simulink model "pv_array"  (R2021a)
settings: Solver=VariableStepAuto  StartTime=0.0  StopTime=10.0  RelTol=1e-3
libraries: spsSeriesRLCBranchLib x2, spsCurrentMeasurementLib x1, spsControlledCurrentSourceLib x1, spsVoltageMeasurementLib x1
settings Model: Creator=Vaneebun  LastModifiedBy=Dell

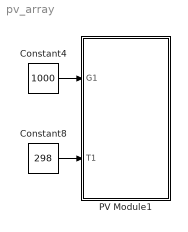
== system pv_array ==
  Constant4 : Constant  Value=1000
  Constant8 : Constant  Value=298
  PV Module1 : Subsystem
  wires:
  Constant8/1 -> PV Module1/2(T1)
  Constant4/1 -> PV Module1/1(G1)

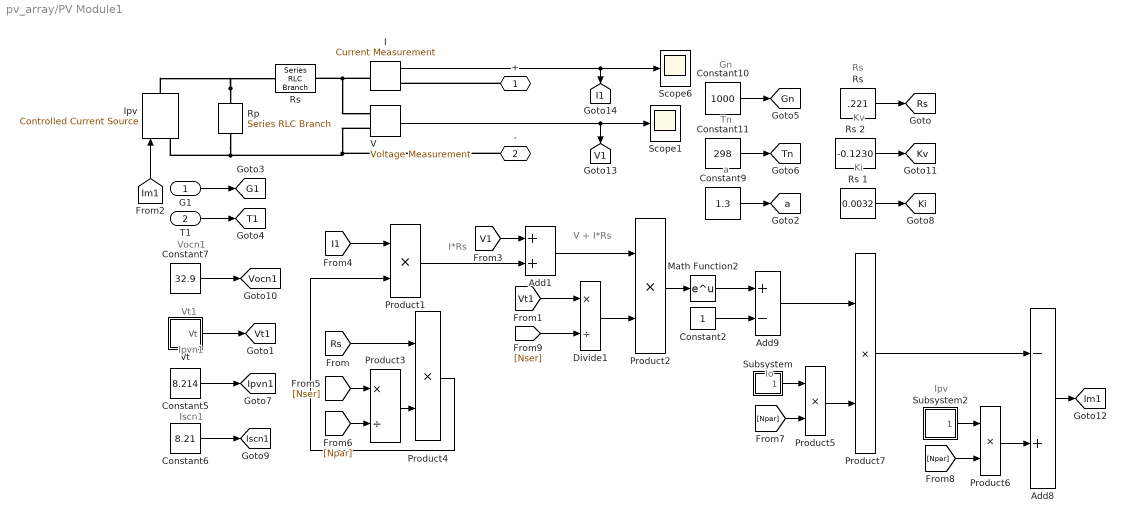
== system pv_array/PV Module1 ==
  note: Vocn1
  note: Iscn1
  note: Ipvn1
  note: I*Rs
  note: Vt1
  note: V + I*Rs
  note: Io
  note: Kv
  note: Ki
  note: Tn
  note: Gn
  note: Rs
  note: a
  note: Ipv
  G1 : Inport
  T1 : Inport  Port=2
  Add1 : Sum
  Add8 : Sum  Inputs=-+
  Add9 : Sum  Inputs=+-
  Constant10 : Constant  Value=1000
  Constant11 : Constant  Value=298
  Constant2 : Constant
  Constant5 : Constant  Value=8.214
  Constant6 : Constant  Value=8.21
  Constant7 : Constant  Value=32.9
  Constant9 : Constant  Value=1.3
  Divide1 : Product  Inputs=*/
  I : spsCurrentMeasurementLib/Current Measurement  PhasorSimulation=off  OutputType=Complex  PSBequivalent=0
  Ipv : spsControlledCurrentSourceLib/Controlled Current Source  Initialize=on  Source_Type=DC  Amplitude=0  Phase=0  Frequency=0  Measurements=None
  Math Function2 : Math  SignedPower=on  SaturateOnIntegerOverflow=on
  Product{1..2,4..7} (6 alike) : Product  RndMeth=Zero
  Product3 : Product  Inputs=*/  RndMeth=Zero
  Rp : spsSeriesRLCBranchLib/Series RLC Branch  LConnTagsString=__new0  RConnTagsString=__new0  BranchType=R  Resistance=3460.32  Inductance=1e-3  SetiL0=off  InitialCurrent=0  Capacitance=1e-6  Setx0=off  InitialVoltage=0  Measurements=None
  Rs : spsSeriesRLCBranchLib/Series RLC Branch  LConnTagsString=__new0  RConnTagsString=__new0  BranchType=R  Resistance=1.84  Inductance=1e-3  SetiL0=off  InitialCurrent=0  Capacitance=1e-6  Setx0=off  InitialVoltage=0  Measurements=None
  "Rs " : Constant  Value=.221
  Rs 1 : Constant  Value=0.0032
  Rs 2 : Constant  Value=-0.1230
  Scope1 : Scope
  Scope6 : Scope
  Subsystem : Subsystem
  Subsystem2 : Subsystem
  "V " : spsVoltageMeasurementLib/Voltage Measurement  PhasorSimulation=off  OutputType=Complex  PSBequivalent=0
  Vt : Subsystem
  + : PMIOPort  Side=Right
  - : PMIOPort  Port=2  Side=Right
  tag scope: G1=global, Gn=global, I1=global, Im1=global, Ipvn1=global, Iscn1=global, Ki=global, Kv=global, Rs=global, T1=global, Tn=global, V1=global, Vocn1=global, Vt1=global, a=global
  wires:
  "V "/1 -> Scope1/1, [V1]
  [I1] -> Product1/1
  [V1] -> Add1/1
  [Im1] -> Ipv/1
  Add8/1 -> [Im1]
  I/1 -> Scope6/1, [I1]
  Product7/1 -> Add8/1
  Add9/1 -> Product7/1
  Constant7/1 -> [Vocn1]
  Constant6/1 -> [Iscn1]
  Constant5/1 -> [Ipvn1]
  T1/1 -> [T1]
  G1/1 -> [G1]
  Vt/1(Vt) -> [Vt1]
  Constant2/1 -> Add9/2
  Math Function2/1 -> Add9/1
  Product2/1 -> Math Function2/1
  Add1/1 -> Product2/1
  Product1/1 -> Add1/2
  Rs 2/1 -> [Kv]
  Rs 1/1 -> [Ki]
  Constant11/1 -> [Tn]
  Constant10/1 -> [Gn]
  Constant9/1 -> [a]
  "Rs "/1 -> [Rs]
  [Nser] -> Product3/1
  [Npar] -> Product3/2
  Product3/1 -> Product4/2
  [Npar] -> Product6/2
  [Rs] -> Product4/1
  Product4/1 -> Product1/2
  Subsystem/1(Out1) -> Product5/1
  [Npar] -> Product5/2
  Product5/1 -> Product7/2
  Subsystem2/1(Out1) -> Product6/1
  Product6/1 -> Add8/2
  [Nser] -> Divide1/2
  [Vt1] -> Divide1/1
  Divide1/1 -> Product2/2
  connections:
  +/RConn1 -- I/RConn1
  "V "/LConn2 -- -/RConn1 -- Rp/RConn1 -- Ipv/LConn1
  Rp/LConn1 -- Ipv/RConn1 -- Rs/LConn1
  I/LConn1 -- Rs/RConn1 -- "V "/LConn1

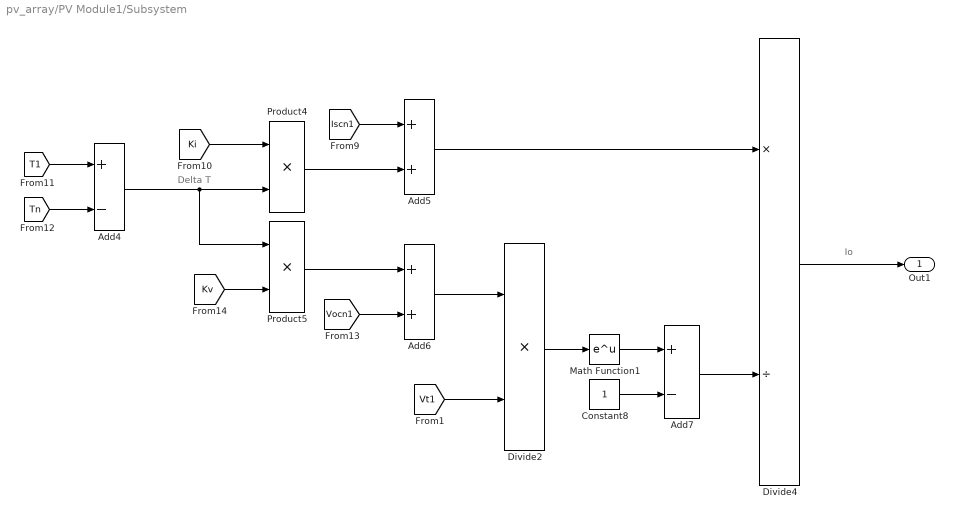
== system pv_array/PV Module1/Subsystem ==
  note: Delta T
  note: Io
  Add4 : Sum  Inputs=+-
  Add5 : Sum
  Add6 : Sum
  Add7 : Sum  Inputs=+-
  Constant8 : Constant
  Divide2 : Product  Inputs=**
  Divide4 : Product  Inputs=*/
  Math Function1 : Math  SignedPower=on  SaturateOnIntegerOverflow=on
  Product4 : Product  RndMeth=Zero
  Product5 : Product  RndMeth=Zero
  Out1 : Outport
  wires:
  [Vt1] -> Divide2/2
  Divide4/1 -> Out1/1
  Add7/1 -> Divide4/2
  Divide2/1 -> Math Function1/1
  Constant8/1 -> Add7/2
  Math Function1/1 -> Add7/1
  Add6/1 -> Divide2/1
  Product5/1 -> Add6/1
  [Kv] -> Product5/2
  [Vocn1] -> Add6/2
  [Tn] -> Add4/2
  Add5/1 -> Divide4/1
  [Iscn1] -> Add5/1
  Product4/1 -> Add5/2
  [Ki] -> Product4/1
  Add4/1 -> Product5/1, Product4/2
  [T1] -> Add4/1

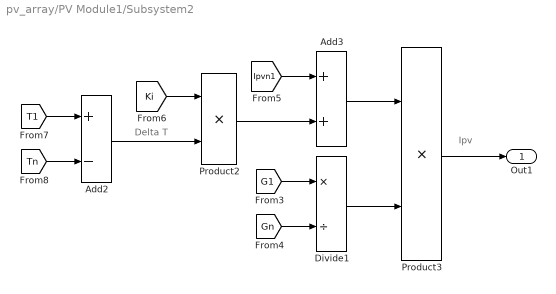
== system pv_array/PV Module1/Subsystem2 ==
  note: Ipv
  note: Delta T
  Add2 : Sum  Inputs=+-
  Add3 : Sum
  Divide1 : Product  Inputs=*/
  Product2 : Product  RndMeth=Zero
  Product3 : Product  RndMeth=Zero
  Out1 : Outport
  wires:
  [G1] -> Divide1/1
  [Gn] -> Divide1/2
  Divide1/1 -> Product3/2
  [Tn] -> Add2/2
  [T1] -> Add2/1
  Add2/1 -> Product2/2
  [Ki] -> Product2/1
  Product2/1 -> Add3/2
  [Ipvn1] -> Add3/1
  Add3/1 -> Product3/1
  Product3/1 -> Out1/1

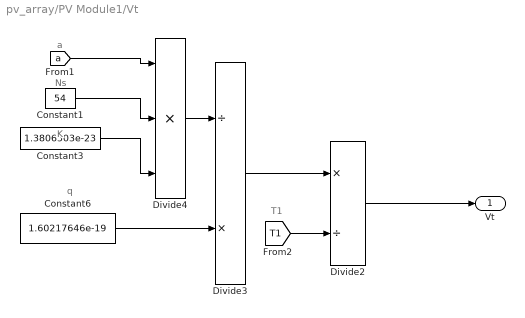
== system pv_array/PV Module1/Vt ==
  note: Ns
  note: K
  note: q
  note: a
  note: T1
  Constant1 : Constant  Value=54
  Constant3 : Constant  Value=1.3806503e-23
  Constant6 : Constant  Value=1.60217646e-19
  Divide2 : Product  Inputs=*/
  Divide3 : Product  Inputs=/*
  Divide4 : Product  Inputs=***
  Vt : Outport
  wires:
  Divide3/1 -> Divide2/1
  Divide4/1 -> Divide3/1
  [T1] -> Divide2/2
  Constant6/1 -> Divide3/2
  Constant3/1 -> Divide4/3
  Constant1/1 -> Divide4/2
  [a] -> Divide4/1
  Divide2/1 -> Vt/1
